simulink model "Task2"  (R2021a)
settings: Solver=FixedStepDiscrete  StartTime=0.0  StopTime=10.0  RelTol=1e-3
settings Model: SILPILModeSetting=veronly  ExtModeTrigDuration=2  Creator=Michael_Ibrahim  LastModifiedBy=Michael_Ibrahim
settings OptimizationCC: EnhancedBackFolding=on  PassReuseOutputArgsAs=Individual arguments  ZeroExternalMemoryAtStartup=off  ZeroInternalMemoryAtStartup=off  MaxStackSize=64  OptimizeBlockOrder=speed  DifferentSizesBufferReuse=on  OptimizationCustomize=off  EfficientTunableParamExpr=on
settings DebuggingCC: UnderspecifiedInitializationDetection=Classic  MergeDetectMultiDrivingBlocksExec=none  ParameterTunabilityLossMsg=error
settings HardwareCC: ProdBitPerInt=16  ProdBitPerPointer=16  ProdBitPerSizeT=16  ProdBitPerPtrDiffT=16  ProdLargestAtomicFloat=None  ProdWordSize=8  ProdHWDeviceType=Atmel->AVR
settings ModelReferenceCC: PropagateSignalLabelsOutOfModel=off
settings SFSimCC: MATLABDynamicMemAlloc=off
settings RTWCC: SystemTargetFile=ert.tlc  HardwareBoard=Arduino Uno  GenCodeOnly=on  TemplateMakefile=ert_default_tmf  GenerateReport=on  Toolchain=Arduino AVR  IncludeHyperlinkInReport=on  LaunchReport=on  GenerateTraceInfo=on  GenerateTraceReport=on  GenerateTraceReportSl=on  GenerateTraceReportSf=on  GenerateTraceReportEml=on
settings CodeAppCC: ForceParamTrailComments=on  IgnoreCustomStorageClasses=off  OperatorAnnotations=on  SimulinkDataObjDesc=on  SFDataObjDesc=on  InsertBlockDesc=on
settings ERTTargetCC: SupportContinuousTime=on  SupportVariableSizeSignals=on  ExtModeStaticAllocSize=250

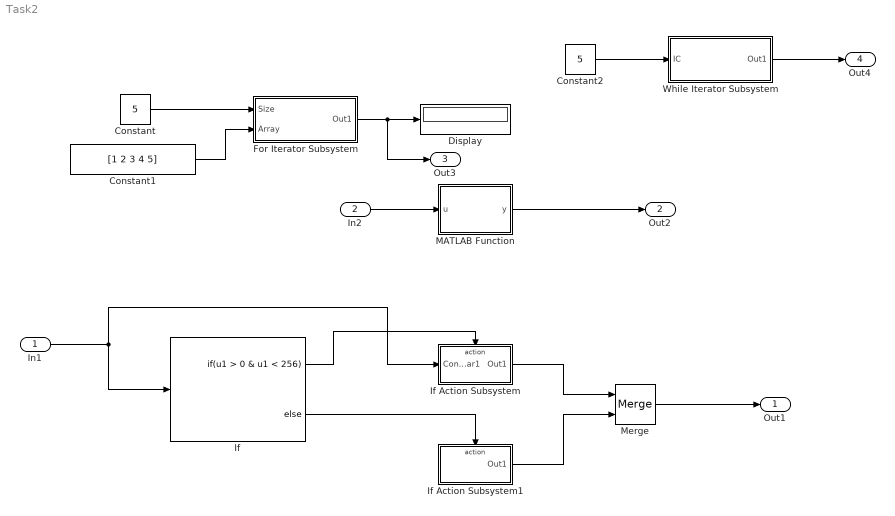
== system Task2 ==
  In1 : Inport
  In2 : Inport  Port=2
  Constant : Constant  Value=5
  Constant1 : Constant  Value=[1 2 3 4 5]
  Constant2 : Constant  Value=5
  Display : Display
  For Iterator Subsystem : Subsystem  TreatAsAtomicUnit=on
  If : If  IfExpression=u1 > 0 & u1 < 256
  If Action Subsystem : Subsystem  TreatAsAtomicUnit=on
  If Action Subsystem1 : Subsystem  TreatAsAtomicUnit=on
  MATLAB Function : MATLAB Function  TreatAsAtomicUnit=on
  Merge : Merge
  While Iterator Subsystem : Subsystem  TreatAsAtomicUnit=on
  Out1 : Outport
  Out2 : Outport  Port=2
  Out3 : Outport  Port=3
  Out4 : Outport  Port=4
  wires:
  If/1 -> If Action Subsystem/Action
  If/2 -> If Action Subsystem1/Action
  In1/1 -> If/1, If Action Subsystem/1(CondPar1)
  If Action Subsystem1/1(Out1) -> Merge/2
  If Action Subsystem/1(Out1) -> Merge/1
  Merge/1 -> Out1/1
  In2/1 -> MATLAB Function/1(u)
  MATLAB Function/1(y) -> Out2/1
  For Iterator Subsystem/1(Out1) -> Out3/1, Display/1
  Constant/1 -> For Iterator Subsystem/1(Size)
  Constant1/1 -> For Iterator Subsystem/2(Array)
  Constant2/1 -> While Iterator Subsystem/1(IC)
  While Iterator Subsystem/1(Out1) -> Out4/1

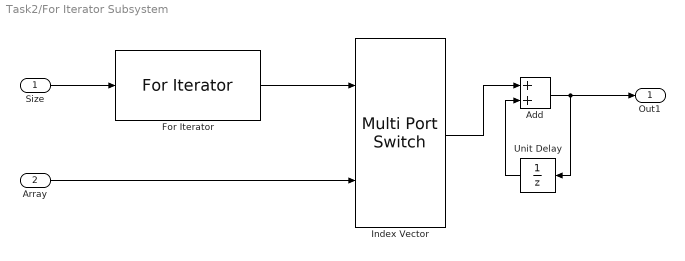
== system Task2/For Iterator Subsystem ==
  Size : Inport
  Array : Inport  Port=2
  Add : Sum
  For Iterator : ForIterator  ResetStates=reset  IterationSource=external  IndexMode=Zero-based
  Index Vector : MultiPortSwitch  DataPortOrder=Zero-based contiguous  Inputs=1  zeroidx=on
  Unit Delay : UnitDelay  SampleTime=-1  HasFrameUpgradeWarning=on
  Out1 : Outport
  wires:
  Index Vector/1 -> Add/1
  Unit Delay/1 -> Add/2
  For Iterator/1 -> Index Vector/1
  Add/1 -> Out1/1, Unit Delay/1
  Size/1 -> For Iterator/1
  Array/1 -> Index Vector/2

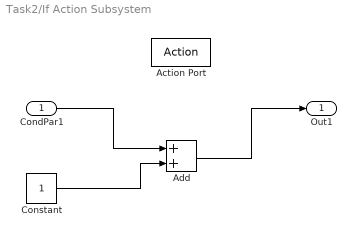
== system Task2/If Action Subsystem ==
  CondPar1 : Inport
  Action Port : ActionPort  ActionPortLabel=if(u1 > 0 & u1 < 256)
  Add : Sum
  Constant : Constant
  Out1 : Outport
  wires:
  CondPar1/1 -> Add/1
  Constant/1 -> Add/2
  Add/1 -> Out1/1

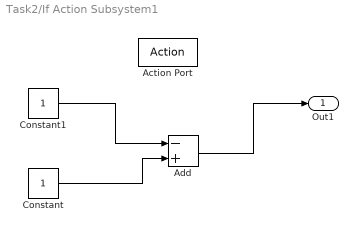
== system Task2/If Action Subsystem1 ==
  Action Port : ActionPort  ActionPortLabel=else
  Add : Sum  Inputs=-+
  Constant : Constant
  Constant1 : Constant
  Out1 : Outport
  wires:
  Constant1/1 -> Add/1
  Constant/1 -> Add/2
  Add/1 -> Out1/1

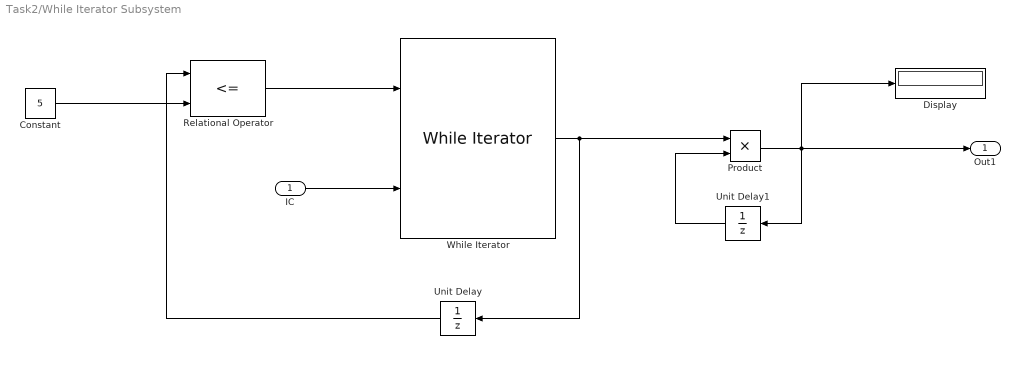
== system Task2/While Iterator Subsystem ==
  IC : Inport
  Constant : Constant  Value=5
  Display : Display
  Product : Product
  Relational Operator : RelationalOperator  Operator=<=  RndMeth=Nearest
  Unit Delay : UnitDelay  InitialCondition=1  SampleTime=-1  HasFrameUpgradeWarning=on
  Unit Delay1 : UnitDelay  InitialCondition=1  SampleTime=-1  HasFrameUpgradeWarning=on
  While Iterator : WhileIterator  ResetStates=reset  ShowIterationPort=on
  Out1 : Outport
  wires:
  IC/1 -> While Iterator/2
  Relational Operator/1 -> While Iterator/1
  Constant/1 -> Relational Operator/2
  Unit Delay/1 -> Relational Operator/1
  While Iterator/1 -> Product/1, Unit Delay/1
  Unit Delay1/1 -> Product/2
  Product/1 -> Unit Delay1/1, Display/1, Out1/1

== matlab function Task2/MATLAB Function ==
  data: u input; y output
function y = fcn(u)
    y = 1;
    for i = 1:u
        y = y * i;
    end
end
